simulink subsystem "non_linear_model"  (R2020a)
settings: Solver=VariableStepAuto  StartTime=0.0  StopTime=10.0  RelTol=1e-3
values from neighbouring files (symbols this model uses):
  g = 9.8    [test.m]    (also in variablen_ersteller.m = 9.81)
  J = 0.001    [variablen_ersteller.m]
  l = 0.3    [test.m]    (also in variablen_ersteller.m = 0.11)
  m = 0.2    [test.m]    (also in variablen_ersteller.m = 0.1756)
  M = 0.5    [test.m]    (also in variablen_ersteller.m = 0.716)
  mue = 0.1    [variablen_ersteller.m]
settings Model: Creator=Alexander Grebien  LastModifiedBy=Alexander Grebien

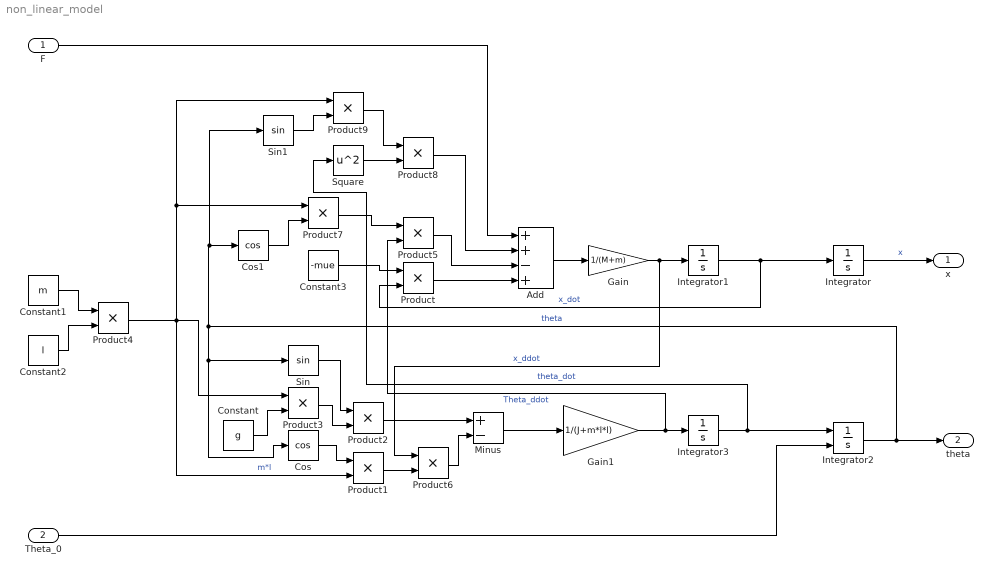
== system non_linear_model ==
  F : Inport
  Theta_0 : Inport  Port=2
  Add : Sum  Inputs=++-+
  Constant : Constant  Value=g
  Constant1 : Constant  Value=m
  Constant2 : Constant  Value=l
  Constant3 : Constant  Value=-mue
  Cos : Trigonometry  Operator=cos
  Cos1 : Trigonometry  Operator=cos
  Gain : Gain  Gain=1/(M+m)
  Gain1 : Gain  Gain=1/(J+m*l*l)
  Integrator : Integrator
  Integrator1 : Integrator
  Integrator2 : Integrator  InitialConditionSource=external
  Integrator3 : Integrator
  Minus : Sum  Inputs=+-
  Product{,1..9} (10 alike) : Product
  Sin : Trigonometry
  Sin1 : Trigonometry
  Square : Math  Operator=square  SaturateOnIntegerOverflow=on
  x : Outport
  theta : Outport  Port=2
  wires:
  Integrator/1 -> x/1  "x"
  Integrator2/1 -> theta/1, Sin1/1, Cos1/1, Sin/1, Cos/1  "theta"
  Add/1 -> Gain/1
  Gain/1 -> Product6/1, Integrator1/1  "x_ddot"
  Gain1/1 -> Integrator3/1, Product5/2  "Theta_ddot"
  Integrator1/1 -> Product/2, Integrator/1  "x_dot"
  Integrator3/1 -> Square/1, Integrator2/1  "theta_dot"
  Minus/1 -> Gain1/1
  Cos/1 -> Product1/1
  Product2/1 -> Minus/1
  Product3/1 -> Product2/2
  Constant/1 -> Product3/2
  Sin/1 -> Product2/1
  Constant1/1 -> Product4/1
  Constant2/1 -> Product4/2
  Product4/1 -> Product9/1, Product7/1, Product1/2, Product3/1  "m*l"
  Product/1 -> Add/4
  Constant3/1 -> Product/1
  Product6/1 -> Minus/2
  Product1/1 -> Product6/2
  Product5/1 -> Add/3
  Product7/1 -> Product5/1
  Cos1/1 -> Product7/2
  Product9/1 -> Product8/1
  Sin1/1 -> Product9/2
  Square/1 -> Product8/2
  Product8/1 -> Add/2
  F/1 -> Add/1
  Theta_0/1 -> Integrator2/2
